simulink model "inversPendulum"  (R2016a)
settings: Solver=VariableStepAuto  StartTime=0.0  StopTime=10  MaxStep=1e-3  MinStep=1e-6  RelTol=1e-5  AbsTol=1e-5
values from neighbouring files (symbols this model uses):
  f_sampling = 30    [parameters.mat]
  g = 9.80665    [parameters.mat]
  l = 0.0825    [parameters.mat]
  m = 0.784    [parameters.mat]
libraries: simulink x1
settings Model: Creator=hda8rt  LastModifiedBy=Adina Haendel
settings SolverCC: InitialStep=1e-4
settings DataIOCC: LimitDataPoints=on
settings DebuggingCC: AllowSymbolicDim=off
settings ModelReferenceCC: PropagateSignalLabelsOutOfModel=off
settings GRTTargetCC: GeneratePreprocessorConditionals=Use local settings

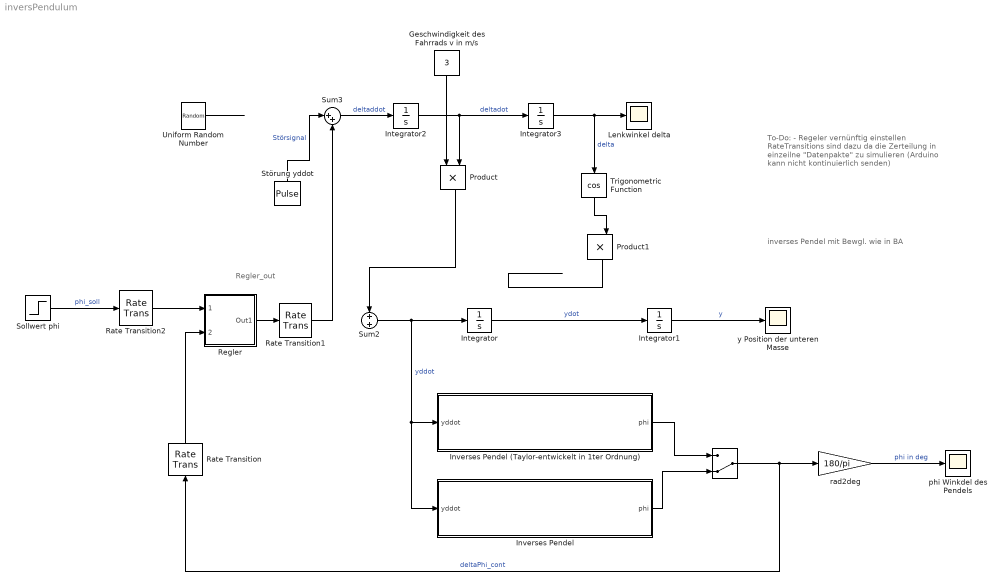
== system inversPendulum ==
  note: Regler_out
  note: To-Do:
      | - Regeler vernünftig einstellen
      |
      | RateTransitions sind dazu da die Zerteilung
      | in einzeilne "Datenpakte" zu simulieren
      | (Arduino kann nicht kontinuierlich senden)
  note: inverses Pendel mit Bewgl. wie in BA
  " " : ManualSwitch  CurrentSetting=0
  Geschwindigkeit des Fahrrads v in m/s : Constant  Value=3
  Integrator{,1..3} (4 alike) : Integrator
  Inverses Pendel : Subsystem
  Inverses Pendel (Taylor-entwickelt in 1ter Ordnung) : Subsystem
  Lenkwinkel delta : Scope
  Product : Product
  Product1 : Product
  Rate Transition : RateTransition  OutPortSampleTime=1/f_sampling
  Rate Transition1 : RateTransition  OutPortSampleTimeOpt=Inherit  OutPortSampleTime=1/f_sampling
  Rate Transition2 : RateTransition  OutPortSampleTime=1/f_sampling
  Regler : Subsystem
  Sollwert phi : Step  Time=20  After=0*pi/180  SampleTime=0
  Störung yddot : DiscretePulseGenerator  PulseType=Time based  Amplitude=2  Period=120  PulseWidth=0.2  PhaseDelay=2
  Sum2 : Sum
  Sum3 : Sum  Inputs=|++
  Trigonometric Function : Trigonometry  Operator=cos
  Uniform Random Number : UniformRandomNumber  SampleTime=0.1
  phi Winkdel des Pendels : Scope
  rad2deg : Gain  Gain=180/pi
  y Position der unteren Masse : Scope
  wires:
  Integrator/1 -> Integrator1/1  "ydot"
  Integrator1/1 -> y Position der unteren Masse/1  "y"
  rad2deg/1 -> phi Winkdel des Pendels/1  "phi in deg"
  Störung yddot/1 -> Sum3/1  "Störsignal"
  Inverses Pendel (Taylor-entwickelt in 1ter Ordnung)/1(phi) -> " "/1
  " "/1 -> Rate Transition/1, rad2deg/1  "deltaPhi_cont"
  Inverses Pendel/1(phi) -> " "/2
  Sum2/1 -> Inverses Pendel/1(yddot), Inverses Pendel (Taylor-entwickelt in 1ter Ordnung)/1(yddot), Integrator/1  "yddot"
  Sollwert phi/1 -> Rate Transition2/1  "phi_soll"
  Regler/1(Out1) -> Rate Transition1/1
  Rate Transition/1 -> Regler/2(phi_ist)
  Rate Transition1/1 -> Sum3/2
  Rate Transition2/1 -> Regler/1(phi_soll)
  Integrator2/1 -> Integrator3/1, Product/2  "deltadot"
  Integrator3/1 -> Trigonometric Function/1, Lenkwinkel delta/1  "delta"
  Geschwindigkeit des Fahrrads v in m/s/1 -> Product/1
  Product/1 -> Sum2/1
  Product1/1 -> ?
  Sum3/1 -> Integrator2/1  "deltaddot"
  Uniform Random Number/1 -> ?
  Trigonometric Function/1 -> Product1/2

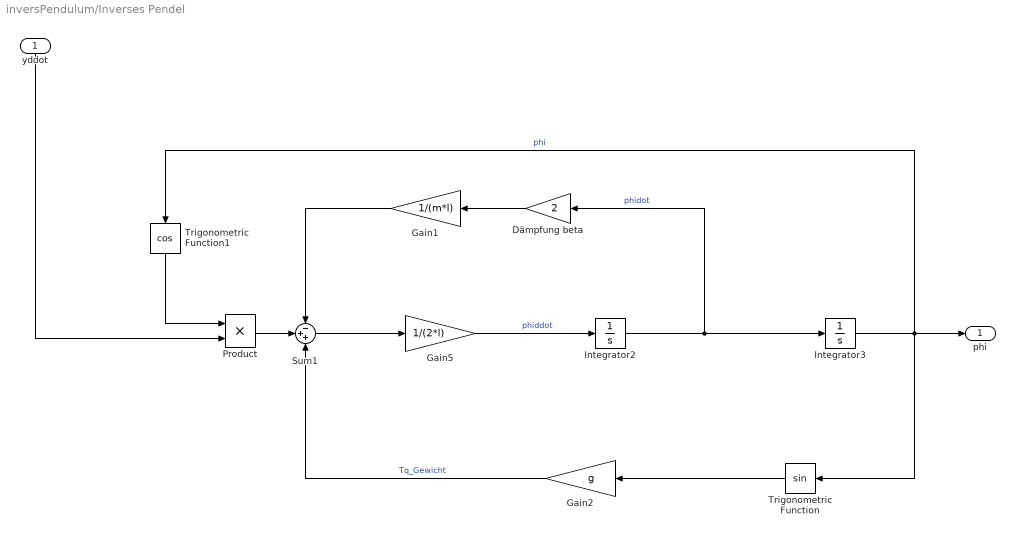
== system inversPendulum/Inverses Pendel ==
  yddot : Inport
  Dämpfung beta : Gain  Gain=2
  Gain1 : Gain  Gain=1/(m*l)
  Gain2 : Gain  Gain=g
  Gain5 : Gain  Gain=1/(2*l)
  Integrator2 : Integrator
  Integrator3 : Integrator  InitialCondition=0*pi/180
  Product : Product  Inputs=**
  Sum1 : Sum  Inputs=-++
  Trigonometric Function : Trigonometry
  Trigonometric Function1 : Trigonometry  Operator=cos
  phi : Outport
  wires:
  Integrator3/1 -> Trigonometric Function1/1, Trigonometric Function/1, phi/1  "phi"
  Gain5/1 -> Integrator2/1  "phiddot"
  Sum1/1 -> Gain5/1
  Integrator2/1 -> Integrator3/1, Dämpfung beta/1  "phidot"
  yddot/1 -> Product/2
  Dämpfung beta/1 -> Gain1/1
  Gain2/1 -> Sum1/3  "Tq_Gewicht"
  Gain1/1 -> Sum1/1
  Trigonometric Function/1 -> Gain2/1
  Trigonometric Function1/1 -> Product/1
  Product/1 -> Sum1/2

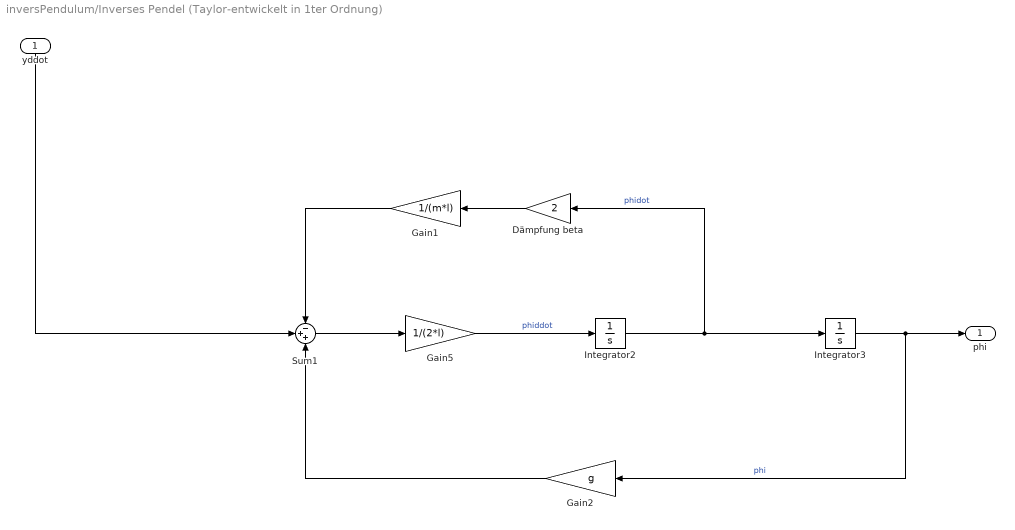
== system inversPendulum/Inverses Pendel (Taylor-entwickelt in 1ter Ordnung) ==
  yddot : Inport
  Dämpfung beta : Gain  Gain=2
  Gain1 : Gain  Gain=1/(m*l)
  Gain2 : Gain  Gain=g
  Gain5 : Gain  Gain=1/(2*l)
  Integrator2 : Integrator
  Integrator3 : Integrator  InitialCondition=0*pi/180
  Sum1 : Sum  Inputs=-++
  phi : Outport
  wires:
  Integrator3/1 -> Gain2/1, phi/1  "phi"
  Gain5/1 -> Integrator2/1  "phiddot"
  Sum1/1 -> Gain5/1
  Integrator2/1 -> Integrator3/1, Dämpfung beta/1  "phidot"
  yddot/1 -> Sum1/2
  Dämpfung beta/1 -> Gain1/1
  Gain2/1 -> Sum1/3
  Gain1/1 -> Sum1/1

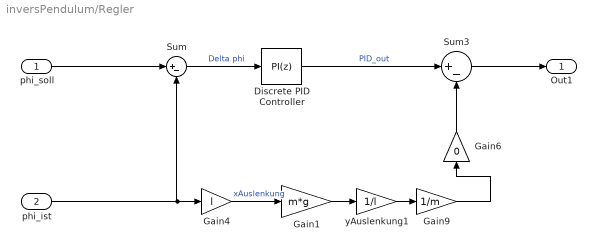
== system inversPendulum/Regler ==
  phi_soll : Inport
  phi_ist : Inport  Port=2
  Discrete PID Controller : simulink/Continuous/PID Controller  Controller=PI  TimeDomain=Discrete-time  SampleTime=-1  IntegratorMethod=Forward Euler  FilterMethod=Forward Euler  Form=Parallel  UseFilter=on  ControllerParametersSource=internal  P=30  I=0  D=0  N=100  InitialConditionSource=internal  InitialConditionForIntegrator=0  InitialConditionForFilter=0  ExternalReset=none  LimitOutput=off  UpperSaturationLimit=inf  LowerSaturationLimit=-inf  LinearizeAsGain=off  AntiWindupMode=none  Kb=1  TrackingMode=off  Kt=1  PParamMin=[]  PParamMax=[]  IParamMin=[]  IParamMax=[]  DParamMin=[]  DParamMax=[]  NParamMin=[]  NParamMax=[]  KbParamMin=[]  KbParamMax=[]  KtParamMin=[]  KtParamMax=[]  POutMin=[]  POutMax=[]  IOutMin=[]  IOutMax=[]  DOutMin=[]  DOutMax=[]  NOutMin=[]  NOutMax=[]  KbOutMin=[]  KbOutMax=[]  KtOutMin=[]  KtOutMax=[]  IntegratorOutMin=[]  IntegratorOutMax=[]  FilterOutMin=[]  FilterOutMax=[]  SumOutMin=[]  SumOutMax=[]  SumI1OutMin=[]  SumI1OutMax=[]  SumI2OutMin=[]  SumI2OutMax=[]  SumI3OutMin=[]  SumI3OutMax=[]  SumDOutMin=[]  SumDOutMax=[]  SaturationOutMin=[]  SaturationOutMax=[]  IntegratorContinuousStateAttributes=''  IntegratorStateMustResolveToSignalObject=off  IntegratorRTWStateStorageClass=Auto  FilterContinuousStateAttributes=''  FilterStateMustResolveToSignalObject=off  FilterRTWStateStorageClass=Auto  DifferentiatorICPrevScaledInput=0  DifferentiatorOutMin=[]  DifferentiatorOutMax=[]
  Gain1 : Gain  Gain=m*g
  Gain4 : Gain  Gain=l
  Gain6 : Gain  Gain=0
  Gain9 : Gain  Gain=1/m
  Sum : Sum  Inputs=|+-
  Sum3 : Sum  Inputs=|+-
  yAuslenkung1 : Gain  Gain=1/l
  Out1 : Outport
  wires:
  Discrete PID Controller/1 -> Sum3/1  "PID_out"
  phi_soll/1 -> Sum/1
  Sum/1 -> Discrete PID Controller/1  "Delta phi"
  Gain4/1 -> Gain1/1  "xAuslenkung"
  Gain1/1 -> yAuslenkung1/1
  yAuslenkung1/1 -> Gain9/1
  Gain9/1 -> Gain6/1
  Gain6/1 -> Sum3/2
  Sum3/1 -> Out1/1
  phi_ist/1 -> Gain4/1, Sum/2
